simulink model "Esm_cur"  (R2025b)
settings: Solver=FixedStepDiscrete  StartTime=0.0  StopTime=0.01  FixedStep=0.001  RelTol=1e-3
settings Model: Creator=leeyj  LastModifiedBy=leeyj

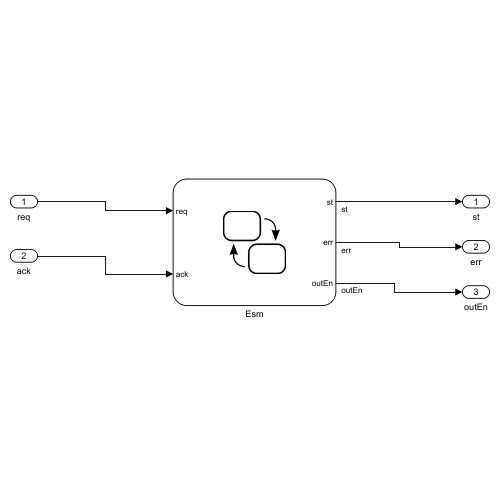
[thumbnail: Simulink's stored preview of the top-level diagram]
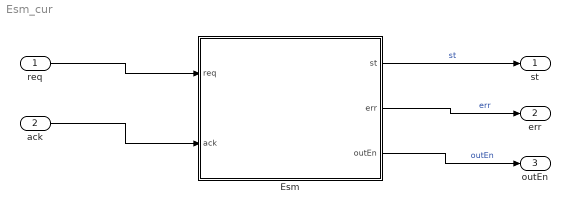
== system Esm_cur ==
  req : Inport  OutDataTypeStr=uint8  Interpolate=off
  ack : Inport  Port=2  OutDataTypeStr=boolean  Interpolate=off
  Esm : Stateflow chart  TreatAsAtomicUnit=on
  st : Outport
  err : Outport  Port=2
  outEn : Outport  Port=3
  wires:
  req/1 -> Esm/1(req)
  ack/1 -> Esm/2(ack)
  Esm/1(st) -> st/1  "st"
  Esm/2(err) -> err/1  "err"
  Esm/3(outEn) -> outEn/1  "outEn"

== stateflow chart Esm_cur/Esm ==
  settings: updateMethod=DISCRETE  sampleTime=0.001
  state Al
    during: err = err && !ack;
    state Init
      entry: st = 1; outEn = false;
      during:
      err = err || (req != 0 && req != st);
    state PreOp
      entry: st = 2; outEn = false;
      during:
      err = err || (req != 0 && req != st);
    state SafeOp
      entry: st = 4; outEn = false;
      during:
      err = err || (req != 0 && req != st);
    state Op
      entry: st = 8; outEn = true;
      during:
      err = err || (req != 0 && req != st);
    (default) -> Init
    Init -> PreOp : [req == 2 && !err]
    PreOp -> SafeOp [order 2] : [req == 4 && !err]
    PreOp -> Init [order 1] : [req == 1]
    SafeOp -> Init [order 1] : [req == 1]
    Op -> Init [order 1] : [req == 1]
    SafeOp -> PreOp [order 2] : [req == 2 && !err]
    Op -> PreOp [order 2] : [req == 2 && !err]
    SafeOp -> Op [order 3] : [req == 8 && !err]
    Op -> SafeOp [order 3] : [req == 4 && !err]
  (default) -> Al
  data: req input uint8; ack input boolean; st output uint8 =1; err output boolean =false; outEn output boolean =false
